simulink model "PID_joint3"  (R2017b)
settings: Solver=VariableStepAuto  StartTime=0.0  StopTime=0.077473  RelTol=1e-3
settings Model: Creator=84935  LastModifiedBy=84935

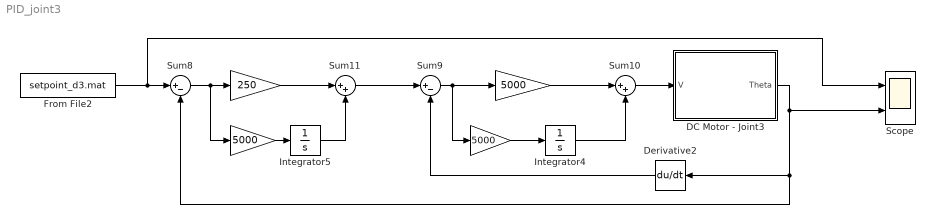
== system PID_joint3 ==
  " " : Gain  Gain=250
  " " : Gain  Gain=5000
  " " : Gain  Gain=5000
  " " : Gain  Gain=5000
  DC Motor - Joint3 : Subsystem  mask{L=0.012342, R=3.2645, Ki=1.1895, Jeff=0.01829, Beff=0.019, Kb=1.1895, N=100}
  Derivative2 : Derivative
  From File2 : FromFile  FileName=setpoint_d3.mat  SampleTime=0
  Integrator4 : Integrator
  Integrator5 : Integrator
  Scope : Scope  NumInputPorts=2
  Sum10 : Sum  Inputs=|++
  Sum11 : Sum  Inputs=|++
  Sum8 : Sum  Inputs=|+-
  Sum9 : Sum  Inputs=|+-
  wires:
  " "/1 -> Integrator4/1
  Sum9/1 -> " "/1, " "/1
  " "/1 -> Sum11/1
  Derivative2/1 -> Sum9/2
  From File2/1 -> Scope/1, Sum8/1
  Integrator4/1 -> Sum10/2
  " "/1 -> Integrator5/1
  Sum11/1 -> Sum9/1
  " "/1 -> Sum10/1
  Integrator5/1 -> Sum11/2
  DC Motor - Joint3/1(Theta) -> Scope/2, Sum8/2, Derivative2/1
  Sum8/1 -> " "/1, " "/1
  Sum10/1 -> DC Motor - Joint3/1(V)

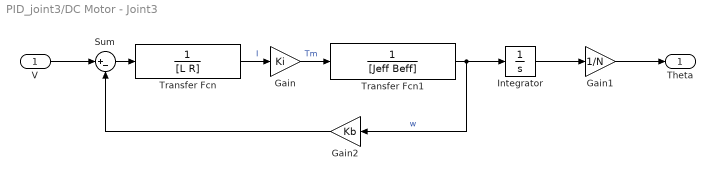
== system PID_joint3/DC Motor - Joint3 ==
  V : Inport
  Gain : Gain  Gain=Ki
  Gain1 : Gain  Gain=1/N
  Gain2 : Gain  Gain=Kb
  Integrator : Integrator
  Sum : Sum  Inputs=|+-
  Transfer Fcn : TransferFcn  Denominator=[L R]
  Transfer Fcn1 : TransferFcn  Denominator=[Jeff Beff]
  Theta : Outport
  wires:
  Integrator/1 -> Gain1/1
  Transfer Fcn1/1 -> Integrator/1, Gain2/1  "w"
  V/1 -> Sum/1
  Gain2/1 -> Sum/2
  Gain/1 -> Transfer Fcn1/1  "Tm"
  Gain1/1 -> Theta/1
  Sum/1 -> Transfer Fcn/1
  Transfer Fcn/1 -> Gain/1  "I"
